simulink model "arduino_android_pedometer_MATLAB_codegen"  (R2025b)
settings: Solver=FixedStepAuto  StartTime=0.0  StopTime=inf  RelTol=1e-3  EnableMultiTasking=on
libraries: arduinowifilib x1
settings Model: SimulationMode=external  ExtModeTrigDuration=2  Creator=The MathWorks, Inc.  LastModifiedBy=The MathWorks, Inc.
settings SolverCC: AlgebraicLoopSolver=TrustRegion
settings DataIOCC: ReturnWorkspaceOutputs=off
settings OptimizationCC: EnhancedBackFolding=on  PassReuseOutputArgsThreshold=0.0  MaxStackSize=64  OptimizeBlockOrder=speed  DifferentSizesBufferReuse=on  OptimizationCustomize=off
settings DebuggingCC: ParameterTunabilityLossMsg=error  UnconnectedInputMsg=warning  UnconnectedOutputMsg=warning  UnconnectedLineMsg=warning  ArithmeticOperatorsInVariantConditions=warning
settings HardwareCC: ProdBitPerPointer=32.0  ProdBitPerSizeT=32.0  ProdBitPerPtrDiffT=32.0  ProdLargestAtomicInteger=Long  ProdLargestAtomicFloat=Double  ProdWordSize=32.0  ProdHWDeviceType=ARM Compatible->ARM Cortex  UseEmbeddedCoderFeatures=off  UseSimulinkCoderFeatures=off
settings ModelReferenceCC: EnableRefExpFcnMdlSchedulingChecks=on
settings SFSimCC: SimUseLocalCustomCode=off  MATLABDynamicMemAlloc=off
settings RTWCC: SystemTargetFile=ert.tlc  HardwareBoard=Arduino MKR1000  TemplateMakefile=ert_default_tmf  GenerateReport=on  RTWUseLocalCustomCode=off  Toolchain=Arduino ARM  BuildConfiguration=Faster Runs  LaunchReport=on  GPUComputeCapability=3.5  DLArmComputeVersion=19.05  Description=Embedded Coder
settings CodeAppCC: ForceParamTrailComments=on  OperatorAnnotations=on
settings ERTTargetCC: ExtModeStaticAllocSize=8192.0  InlinedParameterPlacement=Hierarchical  DynamicArrayContainerType=coder::array  ERTCustomFileBanners=off  SupportContinuousTime=on  SupportNonInlinedSFcns=on  RemoveResetFunc=off  SupportVariableSizeSignals=on  ModelStepFunctionPrototypeControlCompliant=off
settings ConfigComp: CovMetricSettings=dswe

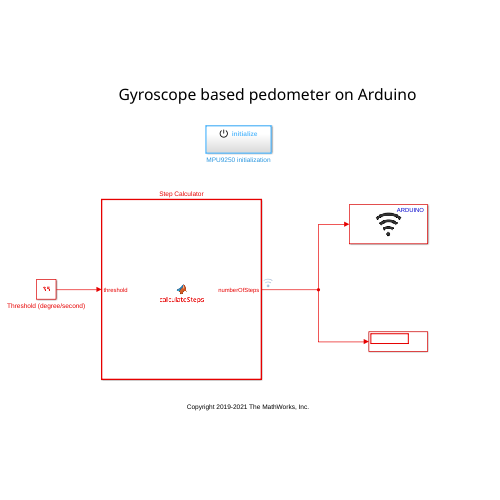
[thumbnail: Simulink's stored preview of the top-level diagram]
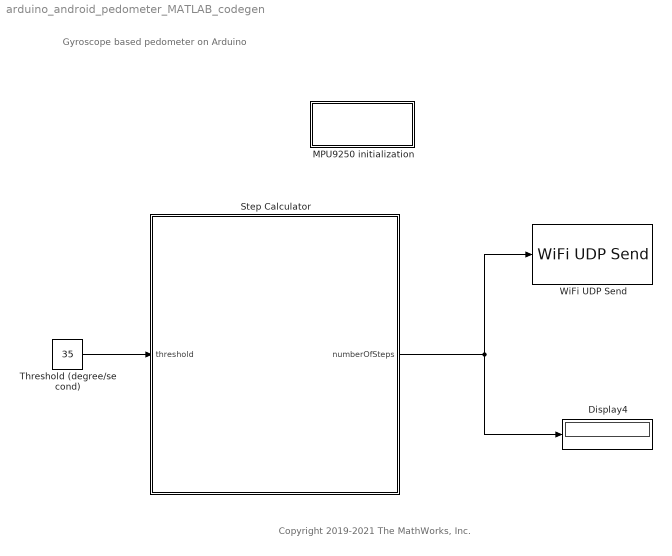
== system arduino_android_pedometer_MATLAB_codegen ==
  note: Copyright 2019-2021 The MathWorks, Inc.
  note: Gyroscope based pedometer on Arduino
  Display4 : Display
  MPU9250 initialization : Subsystem  TreatAsAtomicUnit=on
  Step Calculator : MATLAB Function  TreatAsAtomicUnit=on  SystemSampleTime=1/20
  Threshold (degree/second) : Constant  Value=35  SampleTime=-1
  WiFi UDP Send : arduinowifilib/WiFi UDP Send  remoteIPOctetString=192.168.0.102  remoteport=50002  localport=50001  remoteipoctet1=192  remoteipoctet2=168  remoteipoctet3=0  remoteipoctet4=102  wifiUDPIndex=0  blockPlatform=ARDUINO  isARMArch=true
  wires:
  Step Calculator/1(numberOfSteps) -> WiFi UDP Send/1, Display4/1
  Threshold (degree/second)/1 -> Step Calculator/1(threshold)

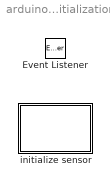
== system arduino_android_pedometer_MATLAB_codegen/MPU9250 initialization ==
  Event Listener : EventListener  DisableCoverage=on  EventName=reset
  initialize sensor : MATLAB Function  TreatAsAtomicUnit=on

== matlab function arduino_android_pedometer_MATLAB_codegen/MPU9250 initialization/initialize sensor ==
function initGyroscope()
% This file initializes the sensor by configuring different registers

% Copyright 2019 The MathWorks, Inc.

PWR_MGMT_1 = hex2dec('6B');
MPU9250_INT_CONFIG = hex2dec('37');
SMPLRT_DIV = hex2dec('19');
CONFIG = hex2dec('1A');
GYRO_CONFIG = hex2dec('1B');

% create arduino hardware and sensor object
arduinoObj = arduino();
gyro = device(arduinoObj, 'I2CAddress', '0x68', 'Bus', 0);

% Configure the sensor
writeRegister(gyro, PWR_MGMT_1, 0);
writeRegister(gyro, MPU9250_INT_CONFIG, 2);
writeRegister(gyro, GYRO_CONFIG, 0);
configVal = readRegister(gyro, CONFIG);
configVal = double(bitor(bitand(configVal, uint8(bin2dec('11111000'))), uint8(bin2dec('00000101'))));
writeRegister(gyro, CONFIG, configVal);
writeRegister(gyro, SMPLRT_DIV, 48);
end

== matlab function arduino_android_pedometer_MATLAB_codegen/Step Calculator ==
  data: numberOfSteps output; threshold input
function numberOfSteps = calculateSteps(threshold)

% This MATLAB function calculates the number of steps taken during a walk
% from the gyroscope readings. The gyroscope must be attached to the leg
% such that the x-axis of the gyroscope lies perpendicular to the leg and
% parallel to the horizontal ground.

% Copyright 2019 The MathWorks, Inc.


persistent steps;
persistent a;
persistent b;
if(isempty(steps))
    steps = uint32(0);
end
numberOfSteps = uint32(steps);
thNegative = -threshold;

%% Read data and frame it
persistent arduinoObj gyroDev;
persistent dataFrame count;
% Length of the frame
frameSize = 50;
% number of data samples from previous frame to be retained in the current
% frame is defined by overlap
overlap = 5;

% Gyroscope register address
gyroDataRegister = hex2dec('43');
gyroResolution = 0.0076;

%% Create arduino and gyroscope sensor object
if isempty(arduinoObj) && isempty(gyroDev)
    arduinoObj = arduino();
    gyroDev = device(arduinoObj, 'I2CAddress', '0x68', 'Bus', 0);
end

%% Read data from the sensor and create a frame
% Read two bytes from the gyroscope register address and convert that into
% double to get current angular velocity
if isempty(count)
    count = 1;
end
if isempty(dataFrame)
    dataFrame = zeros(frameSize, 1);
end
gyroSensorData = readRegister(gyroDev, gyroDataRegister, 2);
gyroData = double((bitor(int16(gyroSensorData(2)), bitshift(int16(gyroSensorData(1)),8))));
gyroData = gyroData*gyroResolution;
if count == 1
    % At the beginning of the frame store last m number of data points from
    % previous frame, where m is defined by overlap
    dataFrame(1:overlap) = dataFrame(end-overlap+1:end);
end
% Put new data in the current frame
dataFrame(overlap+count) = gyroData;
if (overlap+count < frameSize)
    % Do not run the step counting algorithm unless the frame is complete
    count = count + 1;
    return;
else
    % reset the counter once the frame is complete
    count = 1;
end

%% Create a 6th order low pass butterworth filter
% The filter coefficients are fixed and hence calculated only once
fc = coder.const(5);  % Cut-off frequency for the LPF. coder.const is used to avoid creating variables on target
fs = coder.const(20); % Sampling frequency of the filter. It must be same as the sampling frequency of the I2C read block
FilterOrder = coder.const(6);
if(isempty(a))
    [b, a] = butter(FilterOrder, fc/(fs/2));
end

%% Filter the incoming gyro data
filtData = filter(b, a, dataFrame);
secondDerivative = [int8(0); int8(diff(sign(diff(filtData))))];  % 0 is appended allign the index of maxima and minima with the actual data array

%% Find local minimas
minPeakIndex = find(secondDerivative>0);
minPeaks = filtData(minPeakIndex);
minsToBeDiscarded = minPeaks > thNegative;
minPeakIndex(minsToBeDiscarded) = [];
if(isempty(minPeakIndex))
    return;
end

%% Find local maximas
maxPeakIndex = find(secondDerivative<0);
maxPeaks = filtData(maxPeakIndex);
maxToBeDiscarded = maxPeaks < threshold;
maxPeakIndex(maxToBeDiscarded) = [];
if(isempty(maxPeakIndex))
    return;
end

%% Find zero crossings
zeroCrossingIndex = find(diff(sign(filtData)));
if(isempty(zeroCrossingIndex))
    return;
end
if(filtData(zeroCrossingIndex(1)) > 0)
    isNegativeSlope = uint8(1);    % Data starts from a positive value and then crosses zero
else
    isNegativeSlope = uint8(0);    % Data starts from a positive value and then crosses zero
end

%% Calculate number of steps
% After a valid minima, there should be one negative to positive zero
% crossing followed by a valid maxima and vice versa. To avoid false zero
% crossing detection, it must be ensured that a zero crossing is lying
% between one maxima and one minima
i = 1;
while(i <= length(zeroCrossingIndex))
    if(isNegativeSlope)
        if any(find(minPeakIndex > zeroCrossingIndex(i)))
            steps = steps+1;
            currentMinPeakIndex = minPeakIndex(find(minPeakIndex > zeroCrossingIndex(i), 1));
            [row, ~] = find(zeroCrossingIndex > currentMinPeakIndex(1), 1);
            if(~isempty(row))
                row = row(1);    % Ensures scalar value for codegen
                i = row;
            else
                break;
            end
            isNegativeSlope = uint8(0);
        else
            break;
        end
    else
        if any(find(maxPeakIndex > zeroCrossingIndex(i)))
            steps = steps+1;
            currentMaxPeakIndex = maxPeakIndex(find(maxPeakIndex > zeroCrossingIndex(i), 1));
            [row, ~] = find(zeroCrossingIndex > currentMaxPeakIndex(1), 1);
            if(~isempty(row))
                row = row(1);   % Ensures scalar value for codegen
                i = row;
            else
                break;
            end
            isNegativeSlope = uint8(1);
        else
            break;
        end
    end
end
numberOfSteps = steps;
end
